simulink model "non_linear_model_block_simple"  (R2024b)
settings: Solver=FixedStepAuto  StartTime=0.0  StopTime=60  FixedStep=0.1  MaxStep=0.01  RelTol=1e-3
values from neighbouring files (symbols this model uses):
  a = mean(a)    [simulation_parameters_simple.m]
  A_t = 50e2    (= 5000)    [simulation_parameters.m]    (also in simulation_parameters_simple.m = 5e-05)
  K_pump = 1000    [simulation_parameters.m]    (also in simulation_parameters_simple.m = 0.0166666667)
  rho = 997    [simulation_parameters.m]    (also in simulation_parameters_simple.m)
  u0 = 1/4    (= 0.25)    [simulation_parameters.m]    (also in simulation_parameters_simple.m)
libraries: simulink x1, slpidlib x1
settings Model: Creator=andit  LastModifiedBy=andit

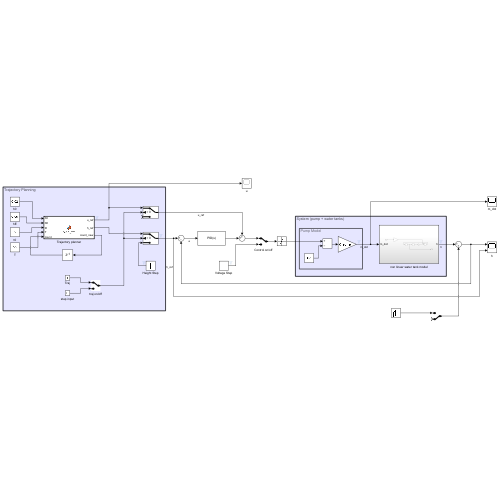
[thumbnail: Simulink's stored preview of the top-level diagram]
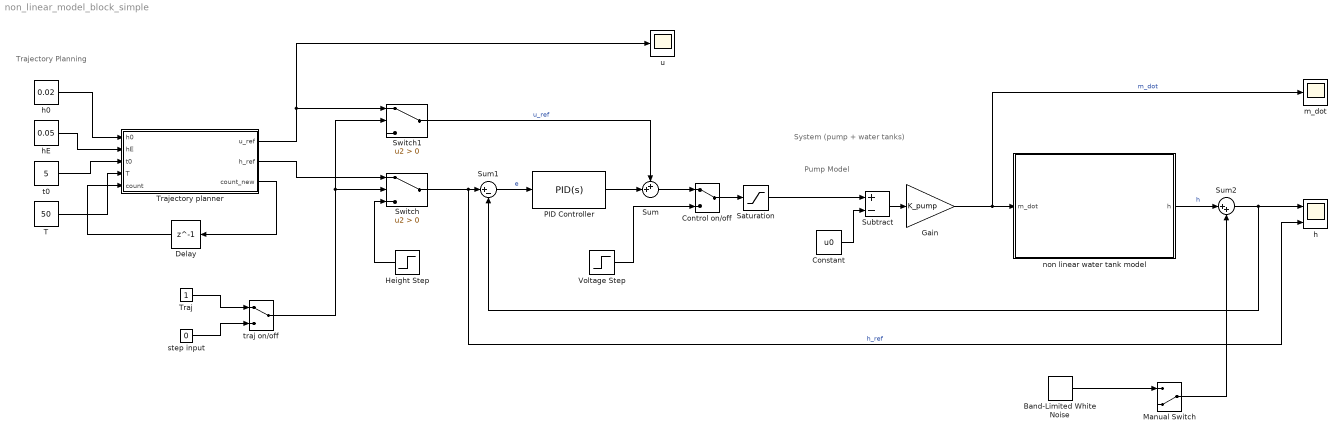
== system non_linear_model_block_simple ==
  note: Trajectory Planning
  note: System (pump + water tanks)
  note: Pump Model
  Band-Limited White Noise : simulink/Sources/Band-Limited White Noise  Cov=[0.00001]  Ts=0.1  seed=[23341]
  Constant : Constant  Value=u0
  Control on/off : ManualSwitch
  Delay : Delay  DelayLength=1
  Gain : Gain  Gain=K_pump
  Height Step : Step  Time=0  Before=0.02  After=0.05  SampleTime=0
  Manual Switch : ManualSwitch  CurrentSetting=0
  PID Controller : slpidlib/PID Controller  Controller=PID  Form=Parallel  TimeDomain=Continuous-time  UseExternalTs=off  SampleTime=-1  IntegratorMethod=Forward Euler  FilterMethod=Forward Euler  ControllerParametersSource=internal  P=0.25637295741853  I=1.97028131388378  UseKiTs=off  D=-0.00242150819674255  UseExternalDerivativeSource=off  N=14.5374139689363  UseFilter=on  TunerSelectOption=Transfer Function Based (PID Tuner App)  InitialConditionSource=internal  InitialConditionForIntegrator=0  InitialConditionForFilter=0  DifferentiatorICPrevScaledInput=0  ExternalReset=none  TrackingMode=off  Kt=1  LimitOutput=off  SatLimitsSource=internal  UpperSaturationLimit=inf  LowerSaturationLimit=-inf  LinearizeAsGain=on  AntiWindupMode=none  Kb=1  LimitIntegrator=off  UpperIntegratorSaturationLimit=inf  LowerIntegratorSaturationLimit=-inf  POutMin=[]  POutMax=[]  IOutMin=[]  IOutMax=[]  DOutMin=[]  DOutMax=[]  NOutMin=[]  NOutMax=[]  SumOutMin=[]  SumOutMax=[]  SaturationOutMin=[]  SaturationOutMax=[]  PParamMin=[]  PParamMax=[]  IParamMin=[]  IParamMax=[]  DParamMin=[]  DParamMax=[]  NParamMin=[]  NParamMax=[]  KbParamMin=[]  KbParamMax=[]  KtParamMin=[]  KtParamMax=[]  KbOutMin=[]  KbOutMax=[]  KtOutMin=[]  KtOutMax=[]  IntegratorOutMin=[]  IntegratorOutMax=[]  FilterOutMin=[]  FilterOutMax=[]  SumI1OutMin=[]  SumI1OutMax=[]  SumI2OutMin=[]  SumI2OutMax=[]  SumI3OutMin=[]  SumI3OutMax=[]  SumI4OutMin=[]  SumI4OutMax=[]  SumDOutMin=[]  SumDOutMax=[]  DifferentiatorOutMin=[]  DifferentiatorOutMax=[]  FilterDiffOutCoefMin=[]  FilterDiffOutCoefMax=[]  ReciprocalOutMin=[]  ReciprocalOutMax=[]  SumDenOutMin=[]  SumDenOutMax=[]  SumNumOutMin=[]  SumNumOutMax=[]  DivideOutMin=[]  DivideOutMax=[]  UdiffTsProdOutMin=[]  UdiffTsProdOutMax=[]  NTsProdOutMin=[]  NTsProdOutMax=[]  UintegralTsProdOutMin=[]  UintegralTsProdOutMax=[]  UngainTsProdOutMin=[]  UngainTsProdOutMax=[]  ClampingZeroOutDataTypeStr=Inherit: Inherit via back propagation  ClampingZeroOutMin=[]  ClampingZeroOutMax=[]  FilterDenConstantOutDataTypeStr=Inherit: Inherit via back propagation  FilterDenConstantOutMin=[]  FilterDenConstantOutMax=[]  PCopyOutDataTypeStr=Inherit: Inherit via back propagation  PCopyOutMin=[]  PCopyOutMax=[]  NCopyOutDataTypeStr=Inherit: Inherit via back propagation  NCopyOutMin=[]  NCopyOutMax=[]  IntegratorContinuousStateAttributes=''  IntegratorStateMustResolveToSignalObject=off  IntegratorRTWStateStorageClass=Auto  FilterContinuousStateAttributes=''  FilterStateMustResolveToSignalObject=off  FilterRTWStateStorageClass=Auto  ParallelPVariant=InternalParameters  IdealPVariant=Disabled  IVariant=InternalParameters  DVariant=InternalParameters  IntegratorVariant=Continuous  SatVariant=Disabled  AWVariant=Passthrough  PCopyVariant=Disabled  TRVariant=Disabled  FdbkBlocksVariant=Forward  IdealPFdbkVariant=Disabled  SatFdbkVariant=Disabled  DerivativeFilterVariant=ContFilter  NVariant=InternalParameters  NCopyVariant=Disabled  FilterICVariant=InternalICsFilter  IntegratorICVariant=InternalICs  ExternalResetVariant=Disabled  TRSumVariant=Passthrough  SumFdbkVariant=Disabled  SumVariant=Sum_PID  TsampFilterVariant=InternalTs  TsampNgainVariant=Passthrough  TsampIntegralVariant=Disabled_SignalSpec  ExternalSaturationOutDataTypeStr=Inherit: Same as second input  DerivativeSourceVariant=ErrorSignal  PreIntVariant=InternalPreInt
  Saturation : Saturate  UpperLimit=5  LowerLimit=0
  Subtract : Sum  Inputs=+-
  Sum : Sum  Inputs=++|
  Sum1 : Sum  Inputs=|+-
  Sum2 : Sum  Inputs=|++
  Switch : Switch  Criteria=u2 > Threshold  SaturateOnIntegerOverflow=off  InputSameDT=off
  Switch1 : Switch  Criteria=u2 > Threshold  SaturateOnIntegerOverflow=off  InputSameDT=off
  T : Constant  Value=50
  Traj : Constant
  Trajectory planner : MATLAB Function  TreatAsAtomicUnit=on
  Voltage Step : Step  After=1.4  SampleTime=0
  h : Scope  NumInputPorts=2
  h0 : Constant  Value=0.02
  hE : Constant  Value=0.05
  m_dot : Scope
  non linear water tank model : Subsystem
  step input : Constant  Value=0
  t0 : Constant  Value=5
  traj on/off : ManualSwitch
  u : Scope
  wires:
  Subtract/1 -> Gain/1
  Constant/1 -> Subtract/2
  Gain/1 -> m_dot/1, non linear water tank model/1(m_dot)  "m_dot"
  PID Controller/1 -> Sum/2
  Sum1/1 -> PID Controller/1  "e"
  Switch/1 -> h/2, Sum1/1  "h_ref"
  Trajectory planner/2(h_ref) -> Switch/1
  traj on/off/1 -> Switch/2, Switch1/2
  Trajectory planner/1(u_ref) -> u/1, Switch1/1
  Switch1/1 -> Sum/1  "u_ref"
  step input/1 -> traj on/off/2
  Traj/1 -> traj on/off/1
  Sum/1 -> Control on/off/1
  h0/1 -> Trajectory planner/1(h0)
  hE/1 -> Trajectory planner/2(hE)
  t0/1 -> Trajectory planner/3(t0)
  T/1 -> Trajectory planner/4(T)
  Trajectory planner/3(count_new) -> Delay/1
  Delay/1 -> Trajectory planner/5(count)
  Control on/off/1 -> Saturation/1
  Saturation/1 -> Subtract/1
  Voltage Step/1 -> Control on/off/2
  Height Step/1 -> Switch/3
  Band-Limited White Noise/1 -> Manual Switch/1
  non linear water tank model/1(h) -> Sum2/1  "h"
  Sum2/1 -> Sum1/2, h/1
  Manual Switch/1 -> Sum2/2

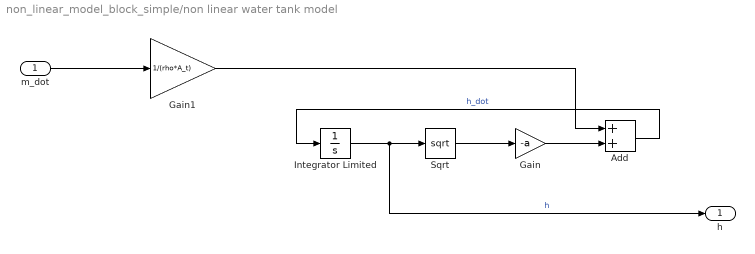
== system non_linear_model_block_simple/non linear water tank model ==
  m_dot : Inport
  Add : Sum
  Gain : Gain  Gain=-a
  Gain1 : Gain  Gain=1/(rho*A_t)
  Integrator Limited : Integrator  InitialCondition=0.02  LimitOutput=on  UpperSaturationLimit=300  LowerSaturationLimit=0
  Sqrt : Sqrt
  h : Outport
  wires:
  Add/1 -> Integrator Limited/1  "h_dot"
  Integrator Limited/1 -> h/1, Sqrt/1  "h"
  Gain/1 -> Add/2
  Sqrt/1 -> Gain/1
  Gain1/1 -> Add/1
  m_dot/1 -> Gain1/1

== matlab function non_linear_model_block_simple/Trajectory planner ==
  data: u_ref output; h_ref output; h0 input; hE input; t0 input; T input; count input; count_new output
function [u_ref, h_ref, count_new] = feed_fw(h0, hE, t0, T, count)

count_new = count+1;
dT = 0.1;
t = count_new*dT-t0;

rho = 997;
A_t = 5e-5; % m^2
K_pump = 0.016666666700000;
u0 = 1/4; % V

a = 1.540430976133678;


x_dot = 0;

if t<0
    x_ref = h0;
elseif t>T
    x_ref = hE;
else
    Dh = hE - h0;
    a0 = h0;
    a1 = 0;
    a2 = 3*Dh / T^2;
    a3 = -2*Dh / T^3;

    x_ref = a0 + a1*t + a2*t^2 + a3*t^3;
    x_dot = a1 + 2*a2*t + 3*a3*t^2;
    
end

h_ref = x_ref;
u_ref = (x_dot + a*sqrt(x_ref))*rho*A_t / (K_pump) + u0; % Sprung im U-ref?
end
